simulink model "DC_Motor_CoastMode"  (R2019b)
settings: Solver=VariableStepAuto  StartTime=0.0  StopTime=10  RelTol=1e-3
PreLoadFcn:
  | modelDir = fileparts(get_param(bdroot, 'FileName'));
  | addpath(fullfile(modelDir,'../../Parameters'));
  | 
  | Parameters_Model
  | Parameters_Simulation
  | Parameters_Controller
InitFcn:
  | Parameters_Model
  | Parameters_Simulation
  | Parameters_Controller
undefined symbols (not defined in the file): B, dTheta0, I0, J, Ke, Kt, L, R, tau_c, theta0
settings Model: Creator=Thomas  LastModifiedBy=thomas.jespersen
settings DataIOCC: ReturnWorkspaceOutputs=off
settings DebuggingCC: ArithmeticOperatorsInVariantConditions=warning
settings SFSimCC: SimUseLocalCustomCode=off  CustomCodeUndefinedFunction=UseInterfaceOnly
settings RTWCC: RTWUseLocalCustomCode=off

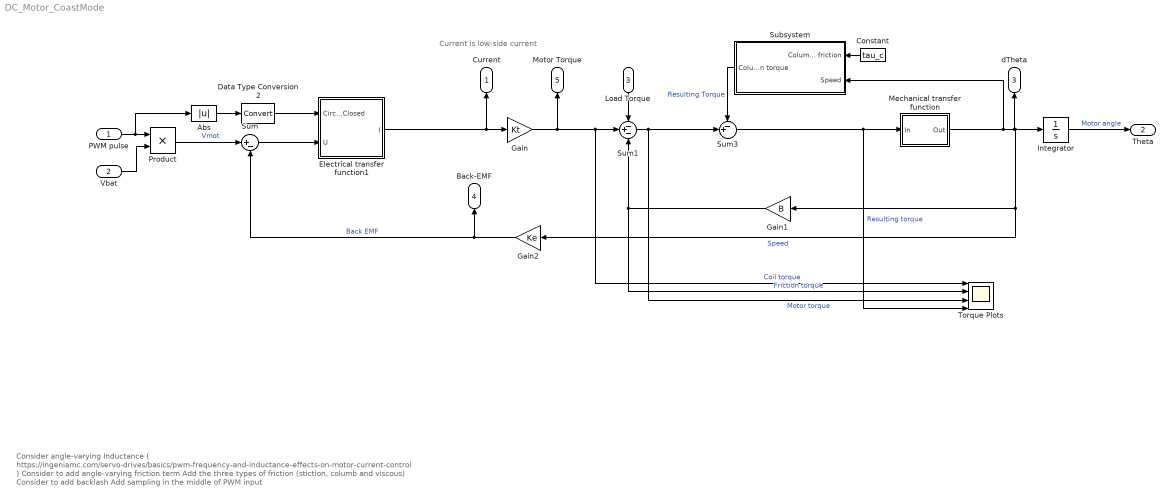
== system DC_Motor_CoastMode ==
  note: Current is low-side current
  note: Consider angle-varying Inductance ( https://ingeniamc.com/servo-drives/basics/pwm-frequency-and-inductance-effects-on-motor-current-control )
      | Consider to add angle-varying friction term
      | Add the three types of friction (stiction, columb and viscous)
      | Consider to add backlash
      | Add sampling in the middle of PWM input
  PWM pulse : Inport  OutDataTypeStr=int8
  Vbat : Inport  Port=2  OutDataTypeStr=double
  Load Torque : Inport  Port=3
  Abs : Abs
  Constant : Constant  Value=tau_c
  Data Type Conversion2 : DataTypeConversion  RndMeth=Round
  Electrical transfer function1 : Subsystem
  Gain : Gain  Gain=Kt
  Gain1 : Gain  Gain=B
  Gain2 : Gain  Gain=Ke
  Integrator : Integrator  InitialCondition=theta0
  Mechanical transfer function : Subsystem
  Product : Product
  Subsystem : Subsystem
  Sum : Sum  Inputs=|+-
  Sum1 : Sum  Inputs=-+-
  Sum3 : Sum  Inputs=-+|
  Torque Plots : Scope  NumInputPorts=4
  Current : Outport  VectorParamsAs1DForOutWhenUnconnected=off
  Theta : Outport  Port=2  VectorParamsAs1DForOutWhenUnconnected=off
  dTheta : Outport  Port=3  VectorParamsAs1DForOutWhenUnconnected=off
  Back-EMF : Outport  Port=4  VectorParamsAs1DForOutWhenUnconnected=off
  Motor Torque : Outport  Port=5  VectorParamsAs1DForOutWhenUnconnected=off
  wires:
  Vbat/1 -> Product/2
  Product/1 -> Sum/1  "Vmot"
  Electrical transfer function1/1(I) -> Current/1, Gain/1
  Sum/1 -> Electrical transfer function1/2(U)
  Gain2/1 -> Back-EMF/1, Sum/2  "Back EMF"
  Load Torque/1 -> Sum1/1
  PWM pulse/1 -> Abs/1, Product/1
  Integrator/1 -> Theta/1  "Motor angle"
  Mechanical transfer function/1(Out) -> Subsystem/2(Speed), Gain1/1, Gain2/1, Integrator/1, dTheta/1  "Speed"
  Sum1/1 -> Torque Plots/3, Sum3/2  "Motor torque"
  Sum3/1 -> Torque Plots/4, Mechanical transfer function/1(In)  "Resulting torque"
  Gain/1 -> Torque Plots/1, Sum1/2, Motor Torque/1  "Coil torque"
  Gain1/1 -> Torque Plots/2, Sum1/3  "Friction torque"
  Data Type Conversion2/1 -> Electrical transfer function1/1(CircuitClosed)
  Abs/1 -> Data Type Conversion2/1
  Constant/1 -> Subsystem/1(Columb friction)
  Subsystem/1(Columb friction torque) -> Sum3/1  "Resulting Torque"

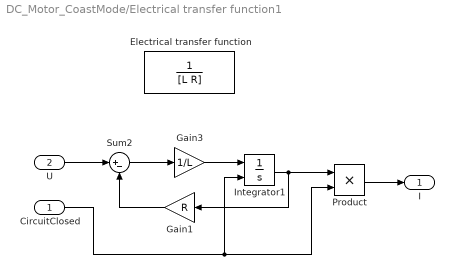
== system DC_Motor_CoastMode/Electrical transfer function1 ==
  CircuitClosed : Inport
  U : Inport  Port=2
  Electrical transfer function : TransferFcn  Denominator=[L R]
  Gain1 : Gain  Gain=R
  Gain3 : Gain  Gain=1/L
  Integrator1 : Integrator  ExternalReset=either  InitialCondition=I0
  Product : Product
  Sum2 : Sum  Inputs=|+-
  I : Outport  VectorParamsAs1DForOutWhenUnconnected=off
  wires:
  U/1 -> Sum2/1
  Gain3/1 -> Integrator1/1
  Gain1/1 -> Sum2/2
  Sum2/1 -> Gain3/1
  Integrator1/1 -> Product/1, Gain1/1
  CircuitClosed/1 -> Product/2, Integrator1/2
  Product/1 -> I/1

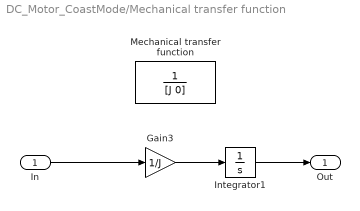
== system DC_Motor_CoastMode/Mechanical transfer function ==
  In : Inport
  Gain3 : Gain  Gain=1/J
  Integrator1 : Integrator  InitialCondition=dTheta0
  Mechanical transfer function : TransferFcn  Denominator=[J 0]
  Out : Outport  VectorParamsAs1DForOutWhenUnconnected=off
  wires:
  Gain3/1 -> Integrator1/1
  In/1 -> Gain3/1
  Integrator1/1 -> Out/1

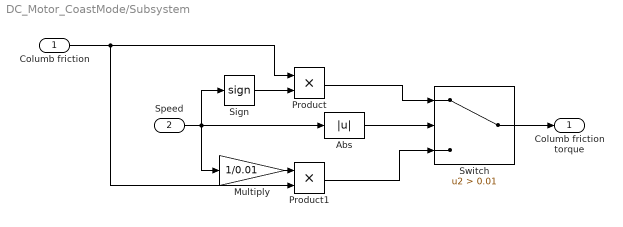
== system DC_Motor_CoastMode/Subsystem ==
  Columb friction : Inport
  Speed : Inport  Port=2  OutDataTypeStr=double
  Abs : Abs
  Multiply : Gain  Gain=1/0.01
  Product : Product
  Product1 : Product
  Sign : Signum
  Switch : Switch  Criteria=u2 > Threshold  Threshold=0.01
  Columb friction torque : Outport  VectorParamsAs1DForOutWhenUnconnected=off
  wires:
  Abs/1 -> Switch/2
  Speed/1 -> Multiply/1, Sign/1, Abs/1
  Sign/1 -> Product/2
  Product/1 -> Switch/1
  Switch/1 -> Columb friction torque/1
  Multiply/1 -> Product1/1
  Product1/1 -> Switch/3
  Columb friction/1 -> Product1/2, Product/1
